simulink model "simple_attitude_controller_FL"  (R2022b)
settings: Solver=ode4  StartTime=0.0  StopTime=5  FixedStep=T_s  RelTol=1e-3
undefined symbols (not defined in the file): A, beta, I_i, m_b, N, prop, rad, s
libraries: slpidlib x4, simulink_extras x3, aerolibconvert2 x1, uavutilslib x1
settings Model: PauseTimes=0.2  Creator=pozzan  LastModifiedBy=pozzan

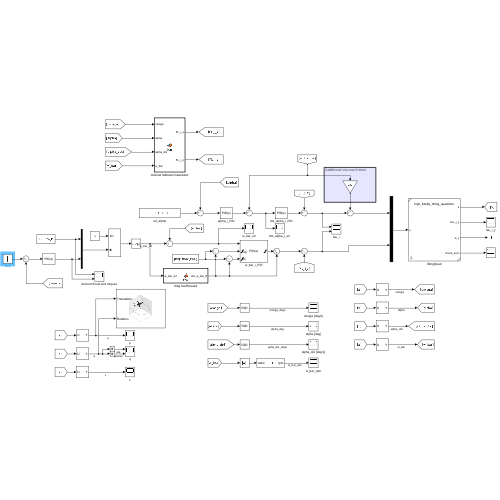
[thumbnail: Simulink's stored preview of the top-level diagram]
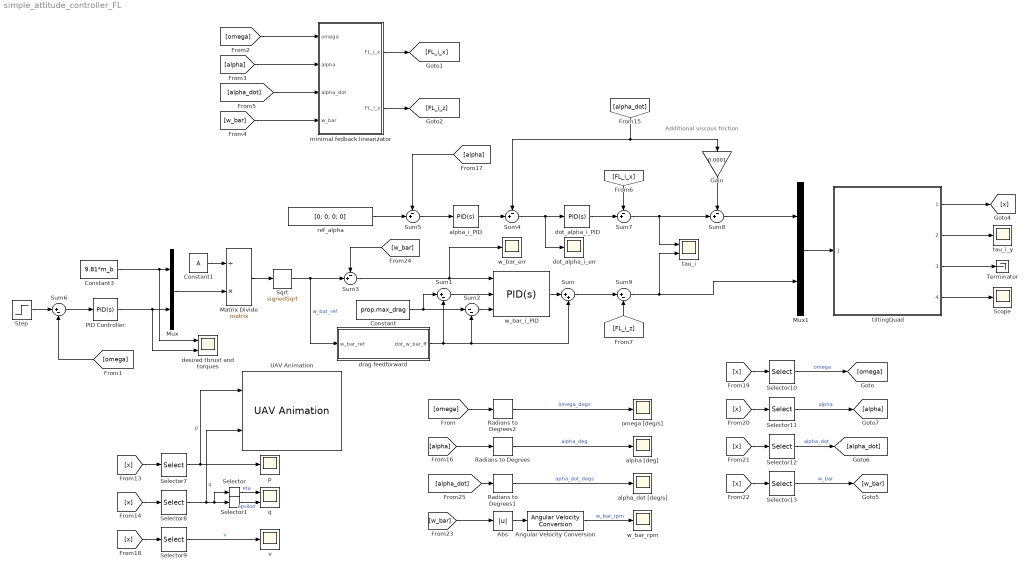
== system simple_attitude_controller_FL ==
  note: Additional viscous friction
  Abs : Abs  SaturateOnIntegerOverflow=off
  Angular Velocity Conversion : aerolibconvert2/Angular Velocity Conversion  IU=rad/s  OU=rpm
  Constant : Constant  Value=prop.max_drag
  Constant1 : Constant  Value=A
  Constant3 : Constant  Value=9.81*m_b  SampleTime=-1
  Gain : Gain  Gain=0.0001
  Matrix Divide : Product  Inputs=/*  Multiplication=Matrix(*)
  Mux : Mux  Inputs=2
  Mux1 : Mux  Inputs=2
  PID Controller : slpidlib/PID Controller  Controller=PID  Form=Parallel  TimeDomain=Continuous-time  UseExternalTs=off  SampleTime=-1  IntegratorMethod=Forward Euler  FilterMethod=Forward Euler  ControllerParametersSource=internal  P=1  I=0.5  UseKiTs=on  D=0  N=100  UseFilter=on  TunerSelectOption=Transfer Function Based (PID Tuner App)  InitialConditionSource=internal  InitialConditionForIntegrator=zeros(3,1)  InitialConditionForFilter=zeros(3,1)  DifferentiatorICPrevScaledInput=0  ExternalReset=none  TrackingMode=off  Kt=1  LimitOutput=off  SatLimitsSource=internal  UpperSaturationLimit=inf  LowerSaturationLimit=-inf  LinearizeAsGain=on  AntiWindupMode=none  Kb=1  LimitIntegrator=off  UpperIntegratorSaturationLimit=inf  LowerIntegratorSaturationLimit=-inf  POutMin=[]  POutMax=[]  IOutMin=[]  IOutMax=[]  DOutMin=[]  DOutMax=[]  NOutMin=[]  NOutMax=[]  SumOutMin=[]  SumOutMax=[]  SaturationOutMin=[]  SaturationOutMax=[]  PParamMin=[]  PParamMax=[]  IParamMin=[]  IParamMax=[]  DParamMin=[]  DParamMax=[]  NParamMin=[]  NParamMax=[]  KbParamMin=[]  KbParamMax=[]  KtParamMin=[]  KtParamMax=[]  KbOutMin=[]  KbOutMax=[]  KtOutMin=[]  KtOutMax=[]  IntegratorOutMin=[]  IntegratorOutMax=[]  FilterOutMin=[]  FilterOutMax=[]  SumI1OutMin=[]  SumI1OutMax=[]  SumI2OutMin=[]  SumI2OutMax=[]  SumI3OutMin=[]  SumI3OutMax=[]  SumI4OutMin=[]  SumI4OutMax=[]  SumDOutMin=[]  SumDOutMax=[]  DifferentiatorOutMin=[]  DifferentiatorOutMax=[]  FilterDiffOutCoefMin=[]  FilterDiffOutCoefMax=[]  ReciprocalOutMin=[]  ReciprocalOutMax=[]  SumDenOutMin=[]  SumDenOutMax=[]  SumNumOutMin=[]  SumNumOutMax=[]  DivideOutMin=[]  DivideOutMax=[]  UdiffTsProdOutMin=[]  UdiffTsProdOutMax=[]  NTsProdOutMin=[]  NTsProdOutMax=[]  UintegralTsProdOutMin=[]  UintegralTsProdOutMax=[]  UngainTsProdOutMin=[]  UngainTsProdOutMax=[]  ClampingZeroOutDataTypeStr=Inherit: Inherit via back propagation  ClampingZeroOutMin=[]  ClampingZeroOutMax=[]  FilterDenConstantOutDataTypeStr=Inherit: Inherit via back propagation  FilterDenConstantOutMin=[]  FilterDenConstantOutMax=[]  PCopyOutDataTypeStr=Inherit: Inherit via back propagation  PCopyOutMin=[]  PCopyOutMax=[]  NCopyOutDataTypeStr=Inherit: Inherit via back propagation  NCopyOutMin=[]  NCopyOutMax=[]  IntegratorContinuousStateAttributes=''  IntegratorStateMustResolveToSignalObject=off  IntegratorRTWStateStorageClass=Auto  FilterContinuousStateAttributes=''  FilterStateMustResolveToSignalObject=off  FilterRTWStateStorageClass=Auto  ParallelPVariant=InternalParameters  IdealPVariant=Disabled  IVariant=InternalParameters  DVariant=InternalParameters  IntegratorVariant=Continuous  SatVariant=Disabled  AWVariant=Passthrough  PCopyVariant=Disabled  TRVariant=Disabled  FdbkBlocksVariant=Forward  IdealPFdbkVariant=Disabled  SatFdbkVariant=Disabled  DerivativeFilterVariant=ContFilter  NVariant=InternalParameters  NCopyVariant=Disabled  FilterICVariant=InternalICsFilter  IntegratorICVariant=InternalICs  ExternalResetVariant=Disabled  TRSumVariant=Passthrough  SumFdbkVariant=Disabled  SumVariant=Sum_PID  TsampFilterVariant=InternalTs  TsampNgainVariant=Passthrough  TsampIntegralVariant=Passthrough  ExternalSaturationOutDataTypeStr=Inherit: Same as second input
  Radians to Degrees : simulink_extras/Transformations/Radians to Degrees
  Radians to Degrees1 : simulink_extras/Transformations/Radians to Degrees
  Radians to Degrees2 : simulink_extras/Transformations/Radians to Degrees
  Scope : Scope
  Selector : Selector  InputPortWidth=4  IndexOptions=Index vector (dialog)  Indices=1  OutputSizes=1
  Selector1 : Selector  InputPortWidth=4  IndexOptions=Index vector (dialog)  Indices=2:4  OutputSizes=1
  Selector10 : Selector  InputPortWidth=13+3*N  IndexOptions=Index vector (dialog)  Indices=11:13  OutputSizes=1
  Selector11 : Selector  InputPortWidth=13+3*N  IndexOptions=Index vector (dialog)  Indices=14:14+N-1  OutputSizes=1
  Selector12 : Selector  InputPortWidth=13+3*N  IndexOptions=Index vector (dialog)  Indices=14+N:14+2*N-1  OutputSizes=1
  Selector13 : Selector  InputPortWidth=13+3*N  IndexOptions=Index vector (dialog)  Indices=14+2*N:14+3*N-1  OutputSizes=1
  Selector7 : Selector  InputPortWidth=13+3*N  IndexOptions=Index vector (dialog)  Indices=1:3  OutputSizes=1
  Selector8 : Selector  InputPortWidth=13+3*N  IndexOptions=Index vector (dialog)  Indices=4:7  OutputSizes=1
  Selector9 : Selector  InputPortWidth=13+3*N  IndexOptions=Index vector (dialog)  Indices=8:10  OutputSizes=1
  Sqrt : Sqrt  Operator=signedSqrt
  Step : Step  Time=2  Before=[1;0;0]  After=[0.00;0;0]  SampleTime=0
  Sum : Sum  Inputs=|++
  Sum1 : Sum  Inputs=|+-
  Sum2 : Sum  Inputs=|--
  Sum{3..5,7..8} (5 alike) : Sum  Inputs=-+|
  Sum6 : Sum  Inputs=|+-
  Sum9 : Sum  Inputs=|+-
  Terminator : Terminator
  UAV Animation : uavutilslib/UAV Animation  UAVType=Multirotor  UAVSize=1  InertialZDirection=Up  SampleTime=0.02
  alpha [deg] : Scope
  alpha_dot [deg/s] : Scope
  alpha_i_PID : slpidlib/PID Controller  Controller=PID  Form=Parallel  TimeDomain=Continuous-time  UseExternalTs=off  SampleTime=-1  IntegratorMethod=Forward Euler  FilterMethod=Forward Euler  ControllerParametersSource=internal  P=75  I=2  UseKiTs=off  D=2  N=100  UseFilter=on  TunerSelectOption=Transfer Function Based (PID Tuner App)  InitialConditionSource=internal  InitialConditionForIntegrator=0  InitialConditionForFilter=0  DifferentiatorICPrevScaledInput=0  ExternalReset=none  TrackingMode=off  Kt=1  LimitOutput=off  SatLimitsSource=internal  UpperSaturationLimit=inf  LowerSaturationLimit=-inf  LinearizeAsGain=on  AntiWindupMode=none  Kb=1  LimitIntegrator=off  UpperIntegratorSaturationLimit=inf  LowerIntegratorSaturationLimit=-inf  POutMin=[]  POutMax=[]  IOutMin=[]  IOutMax=[]  DOutMin=[]  DOutMax=[]  NOutMin=[]  NOutMax=[]  SumOutMin=[]  SumOutMax=[]  SaturationOutMin=[]  SaturationOutMax=[]  PParamMin=[]  PParamMax=[]  IParamMin=[]  IParamMax=[]  DParamMin=[]  DParamMax=[]  NParamMin=[]  NParamMax=[]  KbParamMin=[]  KbParamMax=[]  KtParamMin=[]  KtParamMax=[]  KbOutMin=[]  KbOutMax=[]  KtOutMin=[]  KtOutMax=[]  IntegratorOutMin=[]  IntegratorOutMax=[]  FilterOutMin=[]  FilterOutMax=[]  SumI1OutMin=[]  SumI1OutMax=[]  SumI2OutMin=[]  SumI2OutMax=[]  SumI3OutMin=[]  SumI3OutMax=[]  SumI4OutMin=[]  SumI4OutMax=[]  SumDOutMin=[]  SumDOutMax=[]  DifferentiatorOutMin=[]  DifferentiatorOutMax=[]  FilterDiffOutCoefMin=[]  FilterDiffOutCoefMax=[]  ReciprocalOutMin=[]  ReciprocalOutMax=[]  SumDenOutMin=[]  SumDenOutMax=[]  SumNumOutMin=[]  SumNumOutMax=[]  DivideOutMin=[]  DivideOutMax=[]  UdiffTsProdOutMin=[]  UdiffTsProdOutMax=[]  NTsProdOutMin=[]  NTsProdOutMax=[]  UintegralTsProdOutMin=[]  UintegralTsProdOutMax=[]  UngainTsProdOutMin=[]  UngainTsProdOutMax=[]  ClampingZeroOutDataTypeStr=Inherit: Inherit via back propagation  ClampingZeroOutMin=[]  ClampingZeroOutMax=[]  FilterDenConstantOutDataTypeStr=Inherit: Inherit via back propagation  FilterDenConstantOutMin=[]  FilterDenConstantOutMax=[]  PCopyOutDataTypeStr=Inherit: Inherit via back propagation  PCopyOutMin=[]  PCopyOutMax=[]  NCopyOutDataTypeStr=Inherit: Inherit via back propagation  NCopyOutMin=[]  NCopyOutMax=[]  IntegratorContinuousStateAttributes=''  IntegratorStateMustResolveToSignalObject=off  IntegratorRTWStateStorageClass=Auto  FilterContinuousStateAttributes=''  FilterStateMustResolveToSignalObject=off  FilterRTWStateStorageClass=Auto  ParallelPVariant=InternalParameters  IdealPVariant=Disabled  IVariant=InternalParameters  DVariant=InternalParameters  IntegratorVariant=Continuous  SatVariant=Disabled  AWVariant=Passthrough  PCopyVariant=Disabled  TRVariant=Disabled  FdbkBlocksVariant=Forward  IdealPFdbkVariant=Disabled  SatFdbkVariant=Disabled  DerivativeFilterVariant=ContFilter  NVariant=InternalParameters  NCopyVariant=Disabled  FilterICVariant=InternalICsFilter  IntegratorICVariant=InternalICs  ExternalResetVariant=Disabled  TRSumVariant=Passthrough  SumFdbkVariant=Disabled  SumVariant=Sum_PID  TsampFilterVariant=InternalTs  TsampNgainVariant=Passthrough  TsampIntegralVariant=Passthrough  ExternalSaturationOutDataTypeStr=Inherit: Same as second input
  desired thrust and torques : Scope  NumInputPorts=2
  dot_alpha_i_PID : slpidlib/PID Controller  Controller=PID  Form=Parallel  TimeDomain=Continuous-time  UseExternalTs=off  SampleTime=-1  IntegratorMethod=Forward Euler  FilterMethod=Forward Euler  ControllerParametersSource=internal  P=0.01  I=0.1  UseKiTs=off  D=0.00001  N=100  UseFilter=on  TunerSelectOption=Transfer Function Based (PID Tuner App)  InitialConditionSource=internal  InitialConditionForIntegrator=0  InitialConditionForFilter=0  DifferentiatorICPrevScaledInput=0  ExternalReset=none  TrackingMode=off  Kt=1  LimitOutput=off  SatLimitsSource=internal  UpperSaturationLimit=inf  LowerSaturationLimit=-inf  LinearizeAsGain=on  AntiWindupMode=none  Kb=1  LimitIntegrator=off  UpperIntegratorSaturationLimit=inf  LowerIntegratorSaturationLimit=-inf  POutMin=[]  POutMax=[]  IOutMin=[]  IOutMax=[]  DOutMin=[]  DOutMax=[]  NOutMin=[]  NOutMax=[]  SumOutMin=[]  SumOutMax=[]  SaturationOutMin=[]  SaturationOutMax=[]  PParamMin=[]  PParamMax=[]  IParamMin=[]  IParamMax=[]  DParamMin=[]  DParamMax=[]  NParamMin=[]  NParamMax=[]  KbParamMin=[]  KbParamMax=[]  KtParamMin=[]  KtParamMax=[]  KbOutMin=[]  KbOutMax=[]  KtOutMin=[]  KtOutMax=[]  IntegratorOutMin=[]  IntegratorOutMax=[]  FilterOutMin=[]  FilterOutMax=[]  SumI1OutMin=[]  SumI1OutMax=[]  SumI2OutMin=[]  SumI2OutMax=[]  SumI3OutMin=[]  SumI3OutMax=[]  SumI4OutMin=[]  SumI4OutMax=[]  SumDOutMin=[]  SumDOutMax=[]  DifferentiatorOutMin=[]  DifferentiatorOutMax=[]  FilterDiffOutCoefMin=[]  FilterDiffOutCoefMax=[]  ReciprocalOutMin=[]  ReciprocalOutMax=[]  SumDenOutMin=[]  SumDenOutMax=[]  SumNumOutMin=[]  SumNumOutMax=[]  DivideOutMin=[]  DivideOutMax=[]  UdiffTsProdOutMin=[]  UdiffTsProdOutMax=[]  NTsProdOutMin=[]  NTsProdOutMax=[]  UintegralTsProdOutMin=[]  UintegralTsProdOutMax=[]  UngainTsProdOutMin=[]  UngainTsProdOutMax=[]  ClampingZeroOutDataTypeStr=Inherit: Inherit via back propagation  ClampingZeroOutMin=[]  ClampingZeroOutMax=[]  FilterDenConstantOutDataTypeStr=Inherit: Inherit via back propagation  FilterDenConstantOutMin=[]  FilterDenConstantOutMax=[]  PCopyOutDataTypeStr=Inherit: Inherit via back propagation  PCopyOutMin=[]  PCopyOutMax=[]  NCopyOutDataTypeStr=Inherit: Inherit via back propagation  NCopyOutMin=[]  NCopyOutMax=[]  IntegratorContinuousStateAttributes=''  IntegratorStateMustResolveToSignalObject=off  IntegratorRTWStateStorageClass=Auto  FilterContinuousStateAttributes=''  FilterStateMustResolveToSignalObject=off  FilterRTWStateStorageClass=Auto  ParallelPVariant=InternalParameters  IdealPVariant=Disabled  IVariant=InternalParameters  DVariant=InternalParameters  IntegratorVariant=Continuous  SatVariant=Disabled  AWVariant=Passthrough  PCopyVariant=Disabled  TRVariant=Disabled  FdbkBlocksVariant=Forward  IdealPFdbkVariant=Disabled  SatFdbkVariant=Disabled  DerivativeFilterVariant=ContFilter  NVariant=InternalParameters  NCopyVariant=Disabled  FilterICVariant=InternalICsFilter  IntegratorICVariant=InternalICs  ExternalResetVariant=Disabled  TRSumVariant=Passthrough  SumFdbkVariant=Disabled  SumVariant=Sum_PID  TsampFilterVariant=InternalTs  TsampNgainVariant=Passthrough  TsampIntegralVariant=Passthrough  ExternalSaturationOutDataTypeStr=Inherit: Same as second input
  dot_alpha_i_err : Scope
  drag feedforward : MATLAB Function  TreatAsAtomicUnit=on
  minimal fedback linearizator : MATLAB Function  TreatAsAtomicUnit=on
  omega [deg/s] : Scope
  p : Scope
  q : Scope  NumInputPorts=2
  ref_alpha : Constant  Value=[0; 0; 0; 0]  VectorParams1D=off
  tau_i : Scope  NumInputPorts=2
  tau_i_y : Scope
  tiltingQuad : Subsystem  ReferencedSubsystem=high_fidelity_tilting_quadrotor  p0=p_0  q0=q_0  v0=v_0  omega0=omega_0  alpha0=alpha_0  d_alpha_0=alpha_dot_0  bar_w0=w_bar_0  m_b=m_b  beta=beta  I_b=I_b  I_i=I_i  c_direction=c_direction  k_m=k_m  k_t=k_t  p_mot=p_mot
  v : Scope
  w_bar_err : Scope
  w_bar_i_PID : slpidlib/PID Controller  Controller=PID  Form=Parallel  TimeDomain=Continuous-time  UseExternalTs=off  SampleTime=-1  IntegratorMethod=Forward Euler  FilterMethod=Forward Euler  ControllerParametersSource=internal  P=0.01  I=0.1  UseKiTs=on  D=0.00001  N=100  UseFilter=on  TunerSelectOption=Transfer Function Based (PID Tuner App)  InitialConditionSource=internal  InitialConditionForIntegrator=0  InitialConditionForFilter=0  DifferentiatorICPrevScaledInput=0  ExternalReset=none  TrackingMode=off  Kt=1  LimitOutput=on  SatLimitsSource=external  UpperSaturationLimit=inf  LowerSaturationLimit=-inf  LinearizeAsGain=on  AntiWindupMode=back-calculation  Kb=10  LimitIntegrator=off  UpperIntegratorSaturationLimit=inf  LowerIntegratorSaturationLimit=-inf  POutMin=[]  POutMax=[]  IOutMin=[]  IOutMax=[]  DOutMin=[]  DOutMax=[]  NOutMin=[]  NOutMax=[]  SumOutMin=[]  SumOutMax=[]  SaturationOutMin=[]  SaturationOutMax=[]  PParamMin=[]  PParamMax=[]  IParamMin=[]  IParamMax=[]  DParamMin=[]  DParamMax=[]  NParamMin=[]  NParamMax=[]  KbParamMin=[]  KbParamMax=[]  KtParamMin=[]  KtParamMax=[]  KbOutMin=[]  KbOutMax=[]  KtOutMin=[]  KtOutMax=[]  IntegratorOutMin=[]  IntegratorOutMax=[]  FilterOutMin=[]  FilterOutMax=[]  SumI1OutMin=[]  SumI1OutMax=[]  SumI2OutMin=[]  SumI2OutMax=[]  SumI3OutMin=[]  SumI3OutMax=[]  SumI4OutMin=[]  SumI4OutMax=[]  SumDOutMin=[]  SumDOutMax=[]  DifferentiatorOutMin=[]  DifferentiatorOutMax=[]  FilterDiffOutCoefMin=[]  FilterDiffOutCoefMax=[]  ReciprocalOutMin=[]  ReciprocalOutMax=[]  SumDenOutMin=[]  SumDenOutMax=[]  SumNumOutMin=[]  SumNumOutMax=[]  DivideOutMin=[]  DivideOutMax=[]  UdiffTsProdOutMin=[]  UdiffTsProdOutMax=[]  NTsProdOutMin=[]  NTsProdOutMax=[]  UintegralTsProdOutMin=[]  UintegralTsProdOutMax=[]  UngainTsProdOutMin=[]  UngainTsProdOutMax=[]  ClampingZeroOutDataTypeStr=Inherit: Inherit via back propagation  ClampingZeroOutMin=[]  ClampingZeroOutMax=[]  FilterDenConstantOutDataTypeStr=Inherit: Inherit via back propagation  FilterDenConstantOutMin=[]  FilterDenConstantOutMax=[]  PCopyOutDataTypeStr=Inherit: Inherit via back propagation  PCopyOutMin=[]  PCopyOutMax=[]  NCopyOutDataTypeStr=Inherit: Inherit via back propagation  NCopyOutMin=[]  NCopyOutMax=[]  IntegratorContinuousStateAttributes=''  IntegratorStateMustResolveToSignalObject=off  IntegratorRTWStateStorageClass=Auto  FilterContinuousStateAttributes=''  FilterStateMustResolveToSignalObject=off  FilterRTWStateStorageClass=Auto  ParallelPVariant=InternalParameters  IdealPVariant=Disabled  IVariant=InternalParameters  DVariant=InternalParameters  IntegratorVariant=Continuous  SatVariant=External  AWVariant=BackCalculation  PCopyVariant=Disabled  TRVariant=Disabled  FdbkBlocksVariant=Forward  IdealPFdbkVariant=Disabled  SatFdbkVariant=Disabled  DerivativeFilterVariant=ContFilter  NVariant=InternalParameters  NCopyVariant=Disabled  FilterICVariant=InternalICsFilter  IntegratorICVariant=InternalICs  ExternalResetVariant=Disabled  TRSumVariant=Passthrough  SumFdbkVariant=Disabled  SumVariant=Sum_PID  TsampFilterVariant=InternalTs  TsampNgainVariant=Passthrough  TsampIntegralVariant=Passthrough  ExternalSaturationOutDataTypeStr=Inherit: Same as second input
  w_bar_rpm : Scope
  wires:
  Selector10/1 -> [omega]  "omega"
  [w_bar] -> Abs/1
  Abs/1 -> Angular Velocity Conversion/1
  [x] -> Selector10/1
  [x] -> Selector11/1
  Selector13/1 -> [w_bar]  "w_bar"
  [x] -> Selector7/1
  Selector12/1 -> [alpha_dot]  "alpha_dot"
  Selector9/1 -> v/1  "v"
  [x] -> Selector8/1
  Selector11/1 -> [alpha]  "alpha"
  [alpha] -> Radians to Degrees/1
  Selector7/1 -> UAV Animation/1, p/1  "p"
  [alpha_dot] -> Radians to Degrees1/1
  Selector8/1 -> UAV Animation/2, Selector1/1, Selector/1  "q"
  [x] -> Selector9/1
  [x] -> Selector12/1
  [x] -> Selector13/1
  tiltingQuad/1 -> [x]
  tiltingQuad/2 -> tau_i_y/1
  dot_alpha_i_PID/1 -> Sum7/2
  [w_bar] -> Sum3/1
  Mux1/1 -> tiltingQuad/1
  Sum4/1 -> dot_alpha_i_err/1, dot_alpha_i_PID/1
  ref_alpha/1 -> Sum5/2
  Sum3/1 -> w_bar_err/1, w_bar_i_PID/1
  Sum5/1 -> alpha_i_PID/1
  [alpha_dot] -> Sum4/1, Gain/1
  [alpha] -> Sum5/1
  Selector/1 -> q/1  "eta"
  Selector1/1 -> q/2  "epsilon"
  tiltingQuad/3 -> Terminator/1
  tiltingQuad/4 -> Scope/1
  Radians to Degrees/1 -> alpha [deg]/1  "alpha_deg"
  Radians to Degrees1/1 -> alpha_dot [deg/s]/1  "apha_dot_degs"
  Angular Velocity Conversion/1 -> w_bar_rpm/1  "w_bar_rpm"
  Radians to Degrees2/1 -> omega [deg/s]/1  "omega_degs"
  w_bar_i_PID/1 -> Sum/1
  drag feedforward/1(dot_w_bar_ff) -> Sum/2, Sum2/2, Sum1/2
  Sum1/1 -> w_bar_i_PID/2
  Constant/1 -> Sum2/1, Sum1/1
  Sum2/1 -> w_bar_i_PID/3
  Constant1/1 -> Matrix Divide/1
  Sqrt/1 -> Sum3/2, drag feedforward/1(w_bar_ref)  "w_bar_ref"
  Matrix Divide/1 -> Sqrt/1
  [omega] -> Radians to Degrees2/1
  PID Controller/1 -> desired thrust and torques/2, Mux/2
  Sum6/1 -> PID Controller/1
  Mux/1 -> Matrix Divide/2
  Step/1 -> Sum6/1
  [omega] -> Sum6/2
  Constant3/1 -> desired thrust and torques/1, Mux/1
  Sum7/1 -> tau_i/1, Sum8/2
  Gain/1 -> Sum8/1
  alpha_i_PID/1 -> Sum4/2
  [omega] -> minimal fedback linearizator/1(omega)
  [alpha] -> minimal fedback linearizator/2(alpha)
  [alpha_dot] -> minimal fedback linearizator/3(alpha_dot)
  [w_bar] -> minimal fedback linearizator/4(w_bar)
  minimal fedback linearizator/1(FL_i_x) -> [FL_i_x]
  minimal fedback linearizator/2(FL_i_z) -> [FL_i_z]
  Sum8/1 -> Mux1/1
  [FL_i_x] -> Sum7/1
  Sum9/1 -> tau_i/2, Mux1/2
  [FL_i_z] -> Sum9/2
  Sum/1 -> Sum9/1

== matlab function simple_attitude_controller_FL/minimal fedback linearizator ==
  data: omega input; alpha input; FL_i_x output; beta parameter; N parameter; alpha_dot input; w_bar input; FL_i_z output; I_i parameter
function [FL_i_x, FL_i_z]= fcn(omega, alpha, beta, N, alpha_dot, w_bar, I_i)

FL_i_x = zeros(4,1);
FL_i_z = zeros(4,1);

for i=1:N
    B_R_i = axang2rotm([0 0 1 beta(i)])*axang2rotm([1 0 0 alpha(i)]);
    omega_i = B_R_i.' * omega + [alpha_dot(i); 0; w_bar(i)];
    coriol_i = cross(omega_i, I_i*omega_i);
    FF_i = coriol_i;
    FL_i_x(i) = -FF_i(1);
    FL_i_z(i) = -FF_i(3);
end

== matlab function simple_attitude_controller_FL/drag feedforward ==
  data: w_bar_ref input; dot_w_bar_ff output; k_m parameter
function dot_w_bar_ff = fcn(w_bar_ref, k_m)

dot_w_bar_ff = k_m .* w_bar_ref .* abs(w_bar_ref);
